simulink model "Motor_Param_Est"  (R2014a)
settings: Solver=ode15s  StartTime=0.0  StopTime=4  RelTol=1e-3
PreLoadFcn:
  | load Motor_Param_Est_Data;
PostLoadFcn:
  | open_system([bdroot '/Start Values']);
undefined symbols (not defined in the file): DC_Motor_J
libraries: fl_lib x7, nesl_utility x3, elec_lib x2
Description:
  | Copyright 2014 The MathWorks, Inc.
settings Model: Creator=smiller  LastModifiedBy=psanghvi
settings DataIOCC: ExternalInput=[Motor_Input_time, Motor_Input_Signal]  LoadExternalInput=on
settings OptimizationCC: ExpressionDepthLimit=2147483647  InitFltsAndDblsToZero=on
settings DebuggingCC: UnderspecifiedInitializationDetection=Classic  SolverPrmCheckMsg=none  FcnCallInpInsideContextMsg=UseLocalSettings  StateNameClashWarn=warning
settings GRTTargetCC: CombineOutputUpdateFcns=off  GRTInterface=on

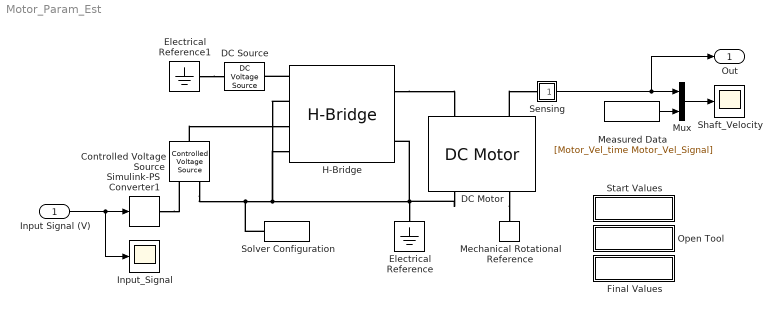
== system Motor_Param_Est ==
  Input Signal (V) : Inport
  Controlled Voltage Source : fl_lib/Electrical/Electrical Sources/Controlled Voltage Source
  DC Motor : elec_lib/Actuators & Drivers/Rotational Actuators/DC Motor  parameterization=1  Ra=DC_Motor_R Ohm  La=DC_Motor_L H  emf_or_torque=1  Kv=DC_Motor_K V/(rad/s)  Ki=6.876e-04 N*m/A  T_stall=2.4e-04 N*m  w_max=4000 rpm  w_rated=2500 rpm  P_rated=10 W  V_rated=12 V  J=DC_Motor_J kg*m^2  lam_param=1  lam=DC_Motor_B N*m/(rad/s)  i_noload=0 A  V_i_noload=1.5 V  speed0=0 rpm  alpha=0.00393 1/K  Tmeas=25 C  thermal_mass=100 J/K  initial_temperature=25 C
  DC Source : fl_lib/Electrical/Electrical Sources/DC Voltage Source  v0=2.5 V
  Electrical Reference : fl_lib/Electrical/Electrical Elements/Electrical Reference
  Electrical Reference1 : fl_lib/Electrical/Electrical Elements/Electrical Reference
  Final Values : Subsystem
      settings: OpenFcn=|
      | DC_Motor_R = 4.0162;
      | DC_Motor_L = 2.0536e-04;
      | DC_Motor_K = 1.0363;
      | DC_Motor_J	 = 0.1306;
      | DC_Motor_B = 1.0630;
      mask Display: disp('Final Values')
  H-Bridge : elec_lib/Actuators & Drivers/Drivers/H-Bridge  Venable=2.5 V  Vmax=5 V  Vreverse=2.5 V  Vbrake=2.5 V  Vm=12 V  pwm_or_av=2  discontinuous=0  freewheeling_mode=1  freewheeling_mode_disc=1  Ron=0.1 Ohm  Don=0.1 Ohm  Rload=10 Ohm  Lload=1e-5 H  F=10 kHz  w_vec=[1, 2] s  i_vec=[1, 2] A  vMatrix=[1, 2; 3, 4] V
  Input_Signal : Scope
      settings: TimeRange=4  YMin=-1  YMax=6  SaveName=DC_Motor_SN_SPE_Input  SampleTime=0.1
  Measured Data : FromWorkspace  VariableName=[Motor_Vel_time Motor_Vel_Signal]  SampleTime=0
  Mechanical Rotational Reference : fl_lib/Mechanical/Rotational Elements/Mechanical Rotational Reference
  Mux : Mux  Inputs=2
  Open Tool : Subsystem
      settings: OpenFcn=speload('Motor_Param_Est_Project', 'Project - Motor_Param_Est', 'Param Est 1');
      mask Display: disp('Open Tool')
  Sensing : Subsystem
      mask Display: disp('S');
  Shaft_Velocity : Scope
      settings: YMin=-1.5  YMax=1.5  SaveName=SS_DC_Motor_SPE_DATA
  Simulink-PS Converter1 : nesl_utility/Simulink-PS Converter  PhysicalDomain=network_engine_domain  SubClassName=ps_input  LeftPortType=input  RightPortType=output  PseudoPeriodic=off  Frequencies=[]  NoiseDistribution=none  NoiseParameters=[]  Unit=1  AffineConversion=off  InputFiltering=off  SimscapeFilterOrder=1  InputFilterTimeConstant=.001  UdotUserProvided=0
  Solver Configuration : nesl_utility/Solver Configuration  PhysicalDomain=network_engine_domain  SubClassName=solver  LeftPortType=input  RightPortType=generic  Accelerate=off  Tones=[]  Harmonics=[]  SimulateNoise=off  Profile=off  UseLocalSampling=off  EnableSwitchedLinearOptims=on  FrequencyDomain=off  UseCCode=off  RelTol=0.001  AbsTol=1e-06  MinStep=1e-09  ToWorkspace=off  DoDC=off  ResidualTolerance=1e-9  UseLocalSolver=off  LocalSolverChoice=NE_BACKWARD_EULER_ADVANCER  LocalSolverSampleTime=.001  DoFixedCost=off  MaxNonlinIter=12  MaxModeIter=2  LinearAlgebra=Sparse  DelaysMemoryBudget=1024  AutomaticFiltering=on  FilteringTimeConstant=0.001
  Start Values : Subsystem
      settings: OpenFcn=|
      | DC_Motor_R = 3;
      | DC_Motor_L = 0.0100;
      | DC_Motor_K = 0.0200;
      | DC_Motor_J	 = 0.0100;
      | DC_Motor_B = 0.5000;
      mask Display: disp('Start Values')
  Out : Outport
  wires:
  Input Signal (V)/1 -> Simulink-PS Converter1/1, Input_Signal/1
  Mux/1 -> Shaft_Velocity/1
  Measured Data/1 -> Mux/2
  Sensing/1(RPM) -> Mux/1, Out/1
  connections:
  DC Motor/RConn2 -- Mechanical Rotational Reference/LConn1
  H-Bridge/LConn1 -- DC Source/LConn1
  Simulink-PS Converter1/RConn1 -- Controlled Voltage Source/RConn1
  Controlled Voltage Source/LConn1 -- H-Bridge/LConn3
  H-Bridge/RConn1 -- DC Motor/LConn1
  Controlled Voltage Source/RConn2 -- Electrical Reference/LConn1 -- H-Bridge/RConn2 -- DC Motor/RConn1 -- H-Bridge/LConn2 -- H-Bridge/LConn4 -- Solver Configuration/RConn1
  Electrical Reference1/LConn1 -- DC Source/RConn1
  DC Motor/LConn2 -- Sensing/LConn1

== system Motor_Param_Est/Final Values ==

== system Motor_Param_Est/Open Tool ==

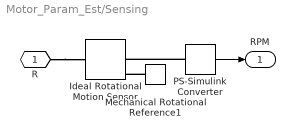
== system Motor_Param_Est/Sensing ==
  Ideal Rotational Motion Sensor : fl_lib/Mechanical/Mechanical Sensors/Ideal Rotational Motion Sensor  offset=0 deg
  Mechanical Rotational Reference1 : fl_lib/Mechanical/Rotational Elements/Mechanical Rotational Reference
  PS-Simulink Converter : nesl_utility/PS-Simulink Converter  PhysicalDomain=network_engine_domain  SubClassName=ps_output  LeftPortType=input  RightPortType=output  PseudoPeriodic=off  Frequencies=[]  Unit=1  AffineConversion=off
  R : PMIOPort  Port=1  Side=Left
  RPM : Outport
  wires:
  PS-Simulink Converter/1 -> RPM/1
  connections:
  PS-Simulink Converter/LConn1 -- Ideal Rotational Motion Sensor/RConn2
  R/RConn1 -- Ideal Rotational Motion Sensor/LConn1
  Mechanical Rotational Reference1/LConn1 -- Ideal Rotational Motion Sensor/RConn1

== system Motor_Param_Est/Start Values ==
